simulink model "compressor_model"  (R2021b)
settings: Solver=ode15s  StartTime=0.0  StopTime=1.5*tsim  MinStep=min_step  RelTol=1e-3  AbsTol=1e-3  EnableMultiTasking=on
InitFcn:
  | warning 'off';
values from neighbouring files (symbols this model uses):
  pc_max = 500e3    (= 500000)    [script_compressor.m]
  R_h2 = 4.12    [script_H2_assumption.m]    (also in script_compressor.m; script_init_pressures.m; script_pipe_dim.m; script_refuel.m)
  Tamb = 273.15+10    (= 283.15)    [script_compressor.m]    (also in script_init_pressures.m; script_pipe_dim.m; script_refuel.m)
  Th2_ref = 273.15-65    (= 208.15)    [script_H2_assumption.m]    (also in script_compressor.m = 283; script_refuel.m = (273.15+15)-20*m)
  tsim = 2000    [script_H2_assumption.m]    (also in script_compressor.m; script_init_pressures.m = 10; script_pipe_dim.m = 30; script_refuel.m)
  vch_o = 0.125    [script_compressor.m]    (also in script_init_pressures.m; script_pipe_dim.m; script_refuel.m)
  ws = 1500    [script_compressor.m]
libraries: fl_lib x50, nesl_utility x6, slpidlib x1, fl_ps_legacy_lib x1
(part 4 of 4)

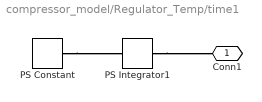
== system compressor_model/Regulator_Temp/time1 ==
  PS Constant : fl_lib/Physical Signals/Sources/PS Constant  constant=1
  PS Integrator1 : fl_lib/Physical Signals/Linear Operators/PS Integrator  reset_method=foundation.enum.IntegratorResetSpec.None  initial_condition_spec=foundation.enum.IntegratorICSpec.Internal  x0=0 s
      settings: SourceProductBaseCode=SS
  Conn1 : PMIOPort  Side=Right
  connections:
  PS Constant/RConn1 -- PS Integrator1/LConn1
  PS Integrator1/RConn1 -- Conn1/RConn1
